simulink model "simSoufflerie_2019a"  (R2019a)
settings: Solver=FixedStepAuto  StartTime=0.0  StopTime=350  FixedStep=0.5  RelTol=1e-3  EnableMultiTasking=on
libraries: mpclib x1
settings Model: Creator=Derick  LastModifiedBy=USER
settings SolverCC: AutoInsertRateTranBlk=on
settings DataIOCC: LimitDataPoints=on  ReturnWorkspaceOutputs=off
settings OptimizationCC: LifeSpan=inf
settings DebuggingCC: SFUnexpectedBacktrackingDiag=warning  SFNoUnconditionalDefaultTransitionDiag=warning  SFExecutionAtInitializationDiag=none  ArithmeticOperatorsInVariantConditions=warning
settings HardwareCC: ProdBitPerSizeT=32  ProdBitPerPtrDiffT=32  ProdWordSize=32  ProdHWDeviceType=Specified
settings ModelReferenceCC: PropagateSignalLabelsOutOfModel=off
settings SFSimCC: SimUseLocalCustomCode=off
settings RTWCC: RTWUseLocalCustomCode=off
settings CodeAppCC: StateflowObjectComments=on
settings GRTTargetCC: TargetLangStandard=C89/C90 (ANSI)
settings ConfigComp: CovMetricSettings=dw  CovHtmlReporting=on  CovSaveCumulativeToWorkspaceVar=on  CovSaveSingleToWorkspaceVar=on  CovExternalEMLEnable=off

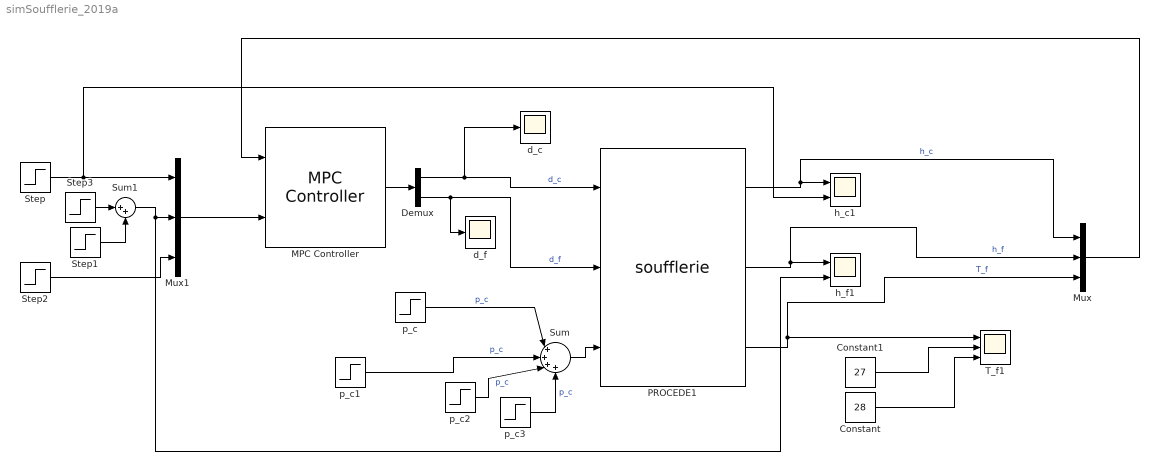
== system simSoufflerie_2019a ==
  Constant : Constant  Value=28
  Constant1 : Constant  Value=27
  Demux : Demux  Outputs=2
  MPC Controller : mpclib/MPC Controller  SCDEnableBlockLinearizationSpecification=on  mpcobj=mpcobj  is_multiple=0  enable_value=0  return_u0=off  updateMPCinCallerWorkspace=on  md_inport=off  mv_inport=off  uref_inport=off  return_cost=off  return_mvseq=off  return_qpstatus=off  return_xseq=off  return_state=off  return_ovseq=off  state_inport=off  umin_inport=off  umax_inport=off  ymin_inport=off  ymax_inport=off  cc_inport=off  ywt_inport=off  uwt_inport=off  duwt_inport=off  rhoeps_inport=off  pm_inport=off  MaximumP=20  HorizonChoice=FixedHorizon  n_ts=0.5  n_p=20  n_mv=2  n_md=0  n_ud=0  n_mo=3  n_uo=0  BlockDataType=double  SampleTimeInherited=off  switch_inport=off
  Mux : Mux  Inputs=3
  Mux1 : Mux  Inputs=3
  PROCEDE1 : M-S-Function  FunctionName=soufflerie
      mask Display:
      | disp('Soufflerie et boucles PI');
      | 
      | port_label('input',1,'d_{csp}','interpreter','tex');
      | port_label('input',2,'d_{fsp}','interpreter','tex');
      | port_label('input',3,'p_{c}','interpreter','tex');
      | 
      | port_label('output',1,'h_{c}','interpreter','tex');
      | port_label('output',2,'h_{f}','interpreter','tex');
      | port_label('output',3,'T_{f}','interpreter','tex');
  Step : Step  Time=150  Before=52.5  After=52.5+25  SampleTime=0
  Step1 : Step  Time=5  Before=51  After=51+10  SampleTime=0
  Step2 : Step  Time=0  After=0  SampleTime=0
  Step3 : Step  Time=150  After=-10  SampleTime=0
  Sum : Sum  Inputs=|++++
  Sum1 : Sum  Inputs=|++
  T_f1 : Scope  NumInputPorts=3
  d_c : Scope
  d_f : Scope
  h_c1 : Scope  NumInputPorts=2
  h_f1 : Scope  NumInputPorts=2
  p_c : Step  Time=50  After=100  SampleTime=0.5
  p_c1 : Step  Time=100  After=-100  SampleTime=0.5
  p_c2 : Step  Time=200  After=100  SampleTime=0.5
  p_c3 : Step  Time=300  After=-100  SampleTime=0.5
  wires:
  Step/1 -> h_c1/2, Mux1/1
  MPC Controller/1 -> Demux/1
  Mux1/1 -> MPC Controller/2
  Mux/1 -> MPC Controller/1
  Demux/2 -> d_f/1, PROCEDE1/2  "d_f"
  PROCEDE1/3 -> Mux/3, T_f1/1  "T_f"
  Demux/1 -> d_c/1, PROCEDE1/1  "d_c"
  Step2/1 -> Mux1/3
  PROCEDE1/2 -> Mux/2, h_f1/1  "h_f"
  PROCEDE1/1 -> Mux/1, h_c1/1  "h_c"
  Sum/1 -> PROCEDE1/3
  Sum1/1 -> h_f1/2, Mux1/2
  Step3/1 -> Sum1/1
  Step1/1 -> Sum1/2
  Constant1/1 -> T_f1/2
  Constant/1 -> T_f1/3
  p_c/1 -> Sum/1  "p_c"
  p_c1/1 -> Sum/2  "p_c"
  p_c2/1 -> Sum/3  "p_c"
  p_c3/1 -> Sum/4  "p_c"
